simulink subsystem "pwm_generator"  (R2022b)
settings: Solver=VariableStepAuto  StartTime=0.0  StopTime=Tsim  RelTol=1e-3
undefined symbols (not defined in the file): SIZE, TYPE
libraries: simulink x6, hdlsllib x2
settings Model: DefaultTestHarness=pwm_generator_harness  Creator=andre  LastModifiedBy=andre
settings ModelReferenceCC: EnableRefExpFcnMdlSchedulingChecks=on

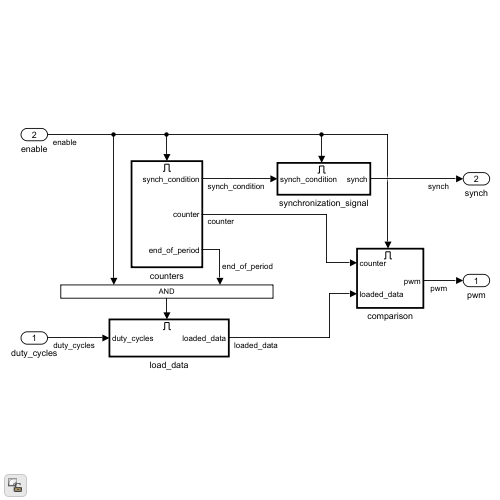
[thumbnail: Simulink's stored preview of the top-level diagram]
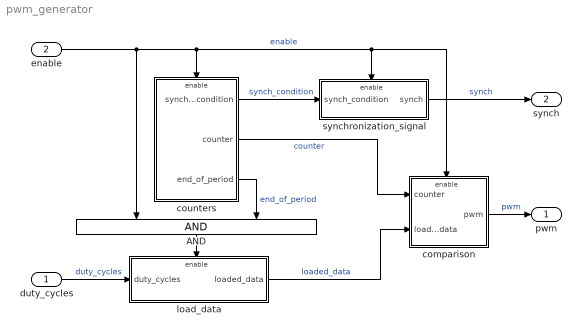
== system pwm_generator ==
  duty_cycles : Inport  OutDataTypeStr=fixdt(0,SIZE,0)  PortDimensions=3
  enable : Inport  Port=2
  AND : Logic  AllPortsSameDT=off  OutDataTypeStr=boolean
  comparison : Subsystem
  counters : Subsystem
  load_data : Subsystem  TreatAsAtomicUnit=on
  synchronization_signal : Subsystem
  pwm : Outport  OutDataTypeStr=boolean  PortDimensions=3
  synch : Outport  Port=2  OutDataTypeStr=boolean  PortDimensions=1
  wires:
  AND/1 -> load_data/Enable
  counters/3(end_of_period) -> AND/2  "end_of_period"
  enable/1 -> AND/1, counters/Enable, comparison/Enable, synchronization_signal/Enable  "enable"
  duty_cycles/1 -> load_data/1(duty_cycles)  "duty_cycles"
  counters/1(synch_condition) -> synchronization_signal/1(synch_condition)  "synch_condition"
  counters/2(counter) -> comparison/1(counter)  "counter"
  load_data/1(loaded_data) -> comparison/2(loaded_data)  "loaded_data"
  synchronization_signal/1(synch) -> synch/1  "synch"
  comparison/1(pwm) -> pwm/1  "pwm"

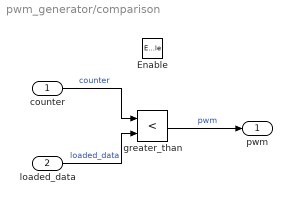
== system pwm_generator/comparison ==
  counter : Inport
  loaded_data : Inport  Port=2
  Enable : EnablePort
  greater_than : RelationalOperator  Operator=<  OutDataTypeStr=boolean  RndMeth=Simplest  InputSameDT=off
  pwm : Outport  InitialOutput=0
  wires:
  loaded_data/1 -> greater_than/2  "loaded_data"
  counter/1 -> greater_than/1  "counter"
  greater_than/1 -> pwm/1  "pwm"

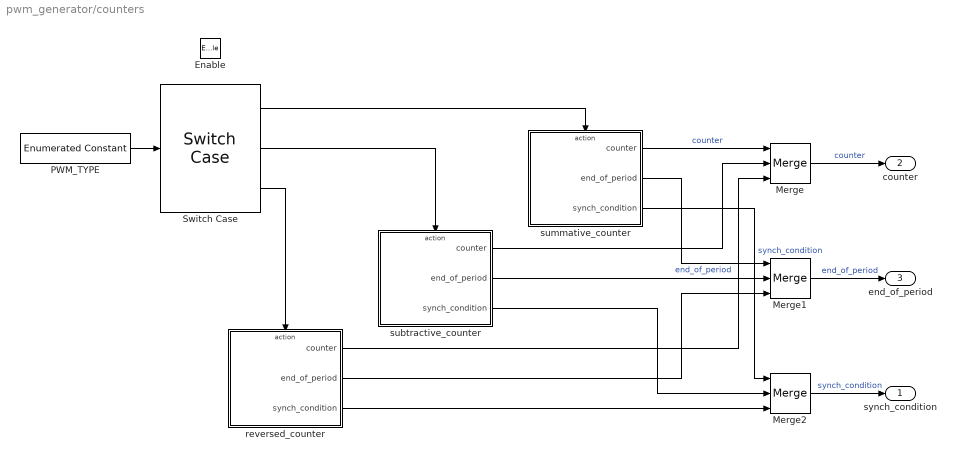
== system pwm_generator/counters ==
  Enable : EnablePort
  Merge : Merge  Inputs=3
  Merge1 : Merge  Inputs=3
  Merge2 : Merge  Inputs=3
  PWM_TYPE : simulink/Sources/Enumerated Constant  OutDataTypeStr=Enum: TYPE  Value=TYPE.FRONT  SampleTime=-1
  Switch Case : SwitchCase  CaseConditions={TYPE.FRONT, TYPE.BACK, TYPE.CENTERED}  ShowDefaultCase=off
  reversed_counter : Subsystem  TreatAsAtomicUnit=on
  subtractive_counter : Subsystem  TreatAsAtomicUnit=on
  summative_counter : Subsystem  TreatAsAtomicUnit=on
  synch_condition : Outport  OutDataTypeStr=boolean  InitialOutput=false
  counter : Outport  Port=2  OutDataTypeStr=fixdt(0,SIZE,0)  InitialOutput=0
  end_of_period : Outport  Port=3  OutDataTypeStr=boolean  InitialOutput=false
  wires:
  Merge2/1 -> synch_condition/1  "synch_condition"
  Merge1/1 -> end_of_period/1  "end_of_period"
  Merge/1 -> counter/1  "counter"
  subtractive_counter/3(synch_condition) -> Merge2/2
  reversed_counter/2(end_of_period) -> Merge1/3
  subtractive_counter/2(end_of_period) -> Merge1/2
  Switch Case/3 -> reversed_counter/Action
  Switch Case/1 -> summative_counter/Action
  subtractive_counter/1(counter) -> Merge/2
  summative_counter/1(counter) -> Merge/1  "counter"
  PWM_TYPE/1 -> Switch Case/1
  reversed_counter/1(counter) -> Merge/3
  Switch Case/2 -> subtractive_counter/Action
  reversed_counter/3(synch_condition) -> Merge2/3
  summative_counter/2(end_of_period) -> Merge1/1  "end_of_period"
  summative_counter/3(synch_condition) -> Merge2/1  "synch_condition"

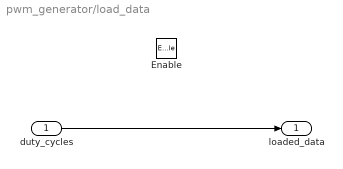
== system pwm_generator/load_data ==
  duty_cycles : Inport
  Enable : EnablePort
  loaded_data : Outport  InitialOutput=0
  wires:
  duty_cycles/1 -> loaded_data/1

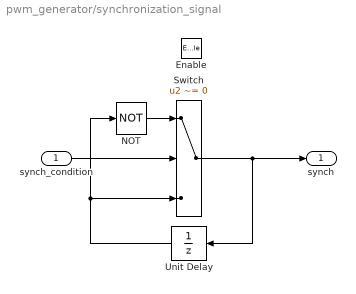
== system pwm_generator/synchronization_signal ==
  synch_condition : Inport
  Enable : EnablePort
  NOT : Logic  Operator=NOT  AllPortsSameDT=off  OutDataTypeStr=boolean
  Switch : Switch  Criteria=u2 ~= 0  SaturateOnIntegerOverflow=off  InputSameDT=off
  Unit Delay : UnitDelay  SampleTime=-1  HasFrameUpgradeWarning=on
  synch : Outport  InitialOutput=0
  wires:
  Unit Delay/1 -> NOT/1, Switch/3
  NOT/1 -> Switch/1
  Switch/1 -> synch/1, Unit Delay/1
  synch_condition/1 -> Switch/2

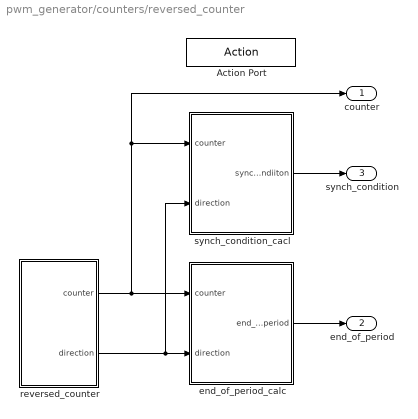
== system pwm_generator/counters/reversed_counter ==
  Action Port : ActionPort
  end_of_period_calc : Subsystem
  reversed_counter : Stateflow chart  TreatAsAtomicUnit=on
  synch_condition_cacl : Subsystem
  counter : Outport  InitialOutput=0
  end_of_period : Outport  Port=2  InitialOutput=0
  synch_condition : Outport  Port=3  InitialOutput=0
  wires:
  reversed_counter/2(direction) -> synch_condition_cacl/2(direction), end_of_period_calc/2(direction)
  end_of_period_calc/1(end_of_period) -> end_of_period/1
  synch_condition_cacl/1(synch_condiiton) -> synch_condition/1
  reversed_counter/1(counter) -> counter/1, synch_condition_cacl/1(counter), end_of_period_calc/1(counter)

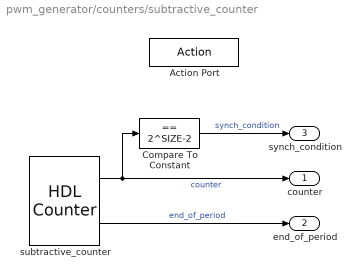
== system pwm_generator/counters/subtractive_counter ==
  Action Port : ActionPort
  Compare To Constant : simulink/Logic and Bit Operations/Compare To Constant  relop===  const=2^SIZE-2  OutDataTypeStr=boolean
  subtractive_counter : hdlsllib/Sources/HDL Counter  CountType=Count limited  CountInit=2^SIZE-2  CountStep=-1  CountMax=0  CountFromType=Initial value  CountFrom=2^SIZE-2  CountResetPort=off  CountLoadPort=off  CountEnbPort=off  CountDirPort=off  CountHitOutputPort=on  CountDataType=Unsigned  CountWordLen=SIZE  CountFracLen=0  CountSampTime=-1
  counter : Outport  InitialOutput=0
  end_of_period : Outport  Port=2  InitialOutput=0
  synch_condition : Outport  Port=3  InitialOutput=0
  wires:
  subtractive_counter/1 -> Compare To Constant/1, counter/1  "counter"
  subtractive_counter/2 -> end_of_period/1  "end_of_period"
  Compare To Constant/1 -> synch_condition/1  "synch_condition"

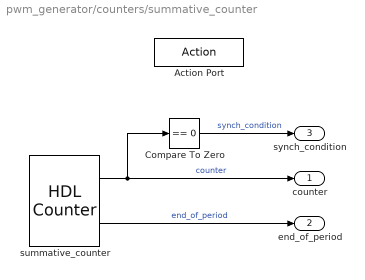
== system pwm_generator/counters/summative_counter ==
  Action Port : ActionPort
  Compare To Zero : simulink/Logic and Bit Operations/Compare To Zero  relop===  OutDataTypeStr=boolean
  summative_counter : hdlsllib/Sources/HDL Counter  CountType=Count limited  CountInit=0  CountStep=1  CountMax=2^SIZE-2  CountFromType=Initial value  CountFrom=0  CountResetPort=off  CountLoadPort=off  CountEnbPort=off  CountDirPort=off  CountHitOutputPort=on  CountDataType=Unsigned  CountWordLen=SIZE  CountFracLen=0  CountSampTime=-1
  counter : Outport  InitialOutput=0
  end_of_period : Outport  Port=2  InitialOutput=0
  synch_condition : Outport  Port=3  InitialOutput=0
  wires:
  Compare To Zero/1 -> synch_condition/1  "synch_condition"
  summative_counter/2 -> end_of_period/1  "end_of_period"
  summative_counter/1 -> Compare To Zero/1, counter/1  "counter"

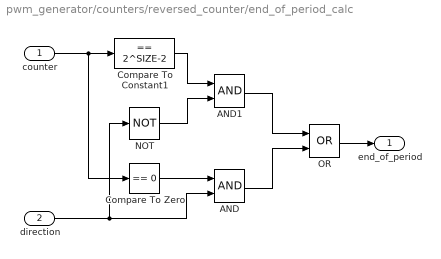
== system pwm_generator/counters/reversed_counter/end_of_period_calc ==
  counter : Inport
  direction : Inport  Port=2
  AND : Logic  AllPortsSameDT=off  OutDataTypeStr=boolean
  AND1 : Logic  AllPortsSameDT=off  OutDataTypeStr=boolean
  Compare To Constant1 : simulink/Logic and Bit Operations/Compare To Constant  relop===  const=2^SIZE-2  OutDataTypeStr=boolean
  Compare To Zero : simulink/Logic and Bit Operations/Compare To Zero  relop===  OutDataTypeStr=boolean
  NOT : Logic  Operator=NOT  AllPortsSameDT=off  OutDataTypeStr=boolean
  OR : Logic  Operator=OR  AllPortsSameDT=off  OutDataTypeStr=boolean
  end_of_period : Outport
  wires:
  AND/1 -> OR/2
  AND1/1 -> OR/1
  direction/1 -> NOT/1, AND/2
  NOT/1 -> AND1/2
  Compare To Zero/1 -> AND/1
  Compare To Constant1/1 -> AND1/1
  counter/1 -> Compare To Zero/1, Compare To Constant1/1
  OR/1 -> end_of_period/1

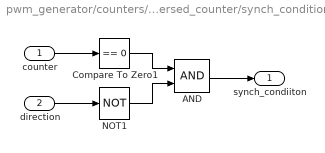
== system pwm_generator/counters/reversed_counter/synch_condition_cacl ==
  counter : Inport
  direction : Inport  Port=2
  AND : Logic  AllPortsSameDT=off  OutDataTypeStr=boolean
  Compare To Zero1 : simulink/Logic and Bit Operations/Compare To Zero  relop===  OutDataTypeStr=boolean
  NOT1 : Logic  Operator=NOT  AllPortsSameDT=off  OutDataTypeStr=boolean
  synch_condiiton : Outport
  wires:
  direction/1 -> NOT1/1
  counter/1 -> Compare To Zero1/1
  Compare To Zero1/1 -> AND/1
  NOT1/1 -> AND/2
  AND/1 -> synch_condiiton/1

== stateflow chart pwm_generator/counters/reversed_counter/reversed_counter ==
  settings: updateMethod=DISCRETE
  state SUMMATIVE
    du:
    counter = fi((counter + fi(1,0,1,0)),0,SIZE,0);
  state SUBTRACTIVE
    du:
    counter = fi((counter - fi(1,0,1,0)),0,SIZE,0);
  (default) -> SUMMATIVE
  SUMMATIVE -> SUBTRACTIVE : [counter == 2^SIZE-2]
      | {direction = true;}
  SUBTRACTIVE -> SUMMATIVE : [counter == 0]
      | {direction = false;}
  data: counter output fixdt(0,SIZE,0) =fi(0,0,SIZE,0); direction output boolean =false; SIZE constant double =SIZE
